simulink model "circuit_Rasp_full_2"  (R2018b)
settings: Solver=VariableStepAuto  StartTime=0.0  StopTime=10.0  RelTol=1e-3
libraries: fl_lib x29, nesl_utility x27, pe_lib x20, elec_lib x6
settings Model: Creator=giovannirenda  LastModifiedBy=giovannirenda
settings DebuggingCC: LibraryContextMissingDiagnostic=none
settings SFSimCC: SimUseLocalCustomCode=off
settings RTWCC: RTWUseLocalCustomCode=off

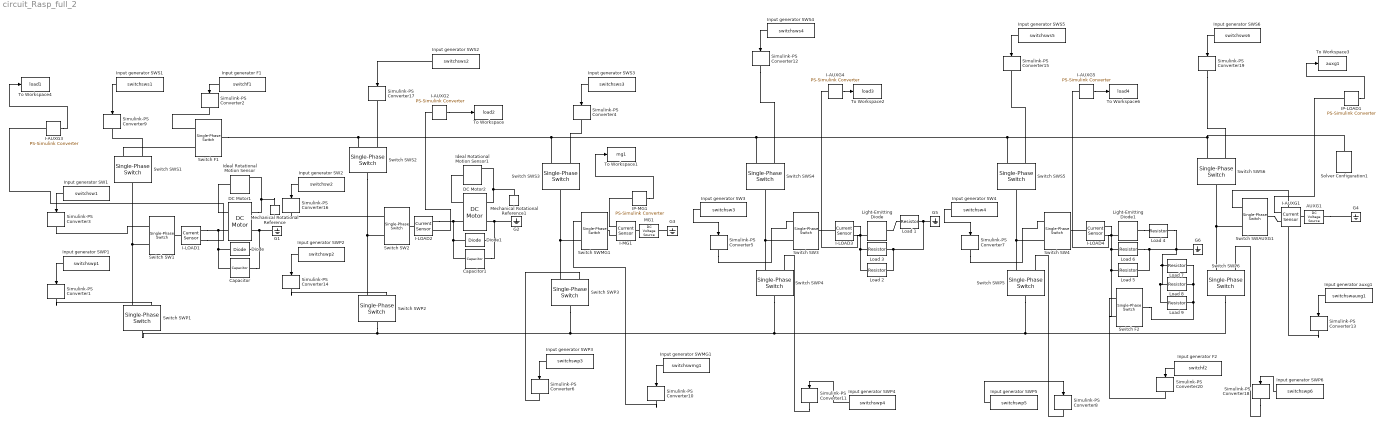
== system circuit_Rasp_full_2 ==
  AUXG1 : fl_lib/Electrical/Electrical Sources/DC Voltage Source  v0=3.3 V
  Capacitor : elec_lib/Passive Devices/Capacitor  enable_table=0  c=10 uF  Cvec=[1e-05, 1e-06] F  Vvec=[0, 10] V  CV_table_symmetry=1  C_tol=5  enable_C_tol=0  tol_distribution=1  nSigma=4  r=1e-6 Ohm  g=0 1/Ohm  enable_operating_limits=0  operating_limit_action=2  max_working_voltage_range=[-25, 25] V  power_rating=1 W  enable_faults=0  fault_action=1  Cscale_faulted=100  R_faulted=1e-3 Ohm  G_faulted=0 1/Ohm  tau_fault=1e-3 s  enable_temporal_fault=0  t_fault=1 s  enable_behavioral_fault=0  max_permissible_voltage_range=[-100, 100] V  t_fail_on_voltage=1 s  i_specify=off  i_priority=None  i=0 A  i_nominal_specify=off  i_nominal_unit=A  i_nominal_value=1  v_specify=off  v_priority=None  v=0 V  v_nominal_specify=off  v_nominal_unit=V  v_nominal_value=1  vc_specify=off  vc_priority=High  vc=0 V  vc_nominal_specify=off  vc_nominal_unit=V  vc_nominal_value=1
  Capacitor1 : elec_lib/Passive Devices/Capacitor  enable_table=0  c=10 uF  Cvec=[1e-05, 1e-06] F  Vvec=[0, 10] V  CV_table_symmetry=1  C_tol=5  enable_C_tol=0  tol_distribution=1  nSigma=4  r=1e-6 Ohm  g=0 1/Ohm  enable_operating_limits=0  operating_limit_action=2  max_working_voltage_range=[-25, 25] V  power_rating=1 W  enable_faults=0  fault_action=1  Cscale_faulted=100  R_faulted=1e-3 Ohm  G_faulted=0 1/Ohm  tau_fault=1e-3 s  enable_temporal_fault=0  t_fault=1 s  enable_behavioral_fault=0  max_permissible_voltage_range=[-100, 100] V  t_fail_on_voltage=1 s  i_specify=off  i_priority=None  i=0 A  i_nominal_specify=off  i_nominal_unit=A  i_nominal_value=1  v_specify=off  v_priority=None  v=0 V  v_nominal_specify=off  v_nominal_unit=V  v_nominal_value=1  vc_specify=off  vc_priority=High  vc=0 V  vc_nominal_specify=off  vc_nominal_unit=V  vc_nominal_value=1
  DC Motor1 : elec_lib/Actuators & Drivers/Rotational Actuators/DC Motor  parameterization=1  Ra=12.7 Ohm  La=12e-6 H  emf_or_torque=1  Kv=0.072e-3 V/rpm  Ki=6.876e-4 N*m/A  T_stall=0.24e-3 N*m  w_max=19100 rpm  w_rated=15000 rpm  P_rated=0.08 W  V_rated=1.5 V  J=0.01 g*cm^2  lam_param=1  lam=0 N*m/(rad/s)  i_noload=0 A  V_i_noload=1.5 V  speed0=0 rpm  alpha=3.93e-3 1/K  Tmeas=25 degC  thermal_mass=100 J/K  initial_temperature=25 degC
  DC Motor2 : elec_lib/Actuators & Drivers/Rotational Actuators/DC Motor  parameterization=1  Ra=12.7 Ohm  La=12e-6 H  emf_or_torque=1  Kv=0.072e-3 V/rpm  Ki=6.876e-4 N*m/A  T_stall=0.24e-3 N*m  w_max=19100 rpm  w_rated=15000 rpm  P_rated=0.08 W  V_rated=1.5 V  J=0.01 g*cm^2  lam_param=1  lam=0 N*m/(rad/s)  i_noload=0 A  V_i_noload=1.5 V  speed0=0 rpm  alpha=3.93e-3 1/K  Tmeas=25 degC  thermal_mass=100 J/K  initial_temperature=25 degC
  Diode : fl_lib/Electrical/Electrical Elements/Diode  Vf=0.6 V  Ron=0.3 Ohm  Goff=1e-8 1/Ohm  i_specify=off  i_priority=None  i=0 A  i_nominal_specify=off  i_nominal_unit=A  i_nominal_value=1  v_specify=off  v_priority=None  v=0 V  v_nominal_specify=off  v_nominal_unit=V  v_nominal_value=1
  Diode1 : fl_lib/Electrical/Electrical Elements/Diode  Vf=0.6 V  Ron=0.3 Ohm  Goff=1e-8 1/Ohm  i_specify=off  i_priority=None  i=0 A  i_nominal_specify=off  i_nominal_unit=A  i_nominal_value=1  v_specify=off  v_priority=None  v=0 V  v_nominal_specify=off  v_nominal_unit=V  v_nominal_value=1
  G{1..6} (6 alike) : fl_lib/Electrical/Electrical Elements/Electrical Reference
  I-AUXG1 : fl_lib/Electrical/Electrical Sensors/Current Sensor
  I-AUXG{2..5} (4 alike) : nesl_utility/PS-Simulink Converter  PhysicalDomain=network_engine_domain  SubClassName=ps_output  LeftPortType=input  RightPortType=output  PseudoPeriodic=off  Frequencies=[]  Unit=A  AffineConversion=off
  I-LOAD{1..4} (4 alike) : fl_lib/Electrical/Electrical Sensors/Current Sensor
  I-MG1 : fl_lib/Electrical/Electrical Sensors/Current Sensor
  IP-LOAD1 : nesl_utility/PS-Simulink Converter  PhysicalDomain=network_engine_domain  SubClassName=ps_output  LeftPortType=input  RightPortType=output  PseudoPeriodic=off  Frequencies=[]  Unit=A  AffineConversion=off
  IP-MG1 : nesl_utility/PS-Simulink Converter  PhysicalDomain=network_engine_domain  SubClassName=ps_output  LeftPortType=input  RightPortType=output  PseudoPeriodic=off  Frequencies=[]  Unit=A  AffineConversion=off
  Ideal Rotational Motion Sensor : fl_lib/Mechanical/Mechanical Sensors/Ideal Rotational Motion Sensor  offset=0 rad
  Ideal Rotational Motion Sensor1 : fl_lib/Mechanical/Mechanical Sensors/Ideal Rotational Motion Sensor  offset=0 rad
  Input generator F1 : FromWorkspace  VariableName=switchf1  SampleTime=1
  Input generator F2 : FromWorkspace  VariableName=switchf2  SampleTime=1
  Input generator SW1 : FromWorkspace  VariableName=switchsw1  SampleTime=1
  Input generator SW2 : FromWorkspace  VariableName=switchsw2  SampleTime=1
  Input generator SW3 : FromWorkspace  VariableName=switchsw3  SampleTime=1
  Input generator SW4 : FromWorkspace  VariableName=switchsw4  SampleTime=1
  Input generator SWMG1 : FromWorkspace  VariableName=switchswmg1  SampleTime=1
  Input generator SWP1 : FromWorkspace  VariableName=switchswp1  SampleTime=1
  Input generator SWP2 : FromWorkspace  VariableName=switchswp2  SampleTime=1
  Input generator SWP3 : FromWorkspace  VariableName=switchswp3  SampleTime=1
  Input generator SWP4 : FromWorkspace  VariableName=switchswp4  SampleTime=1
  Input generator SWP5 : FromWorkspace  VariableName=switchswp5  SampleTime=1
  Input generator SWP6 : FromWorkspace  VariableName=switchswp6  SampleTime=1
  Input generator SWS1 : FromWorkspace  VariableName=switchsws1  SampleTime=1
  Input generator SWS2 : FromWorkspace  VariableName=switchsws2  SampleTime=1
  Input generator SWS3 : FromWorkspace  VariableName=switchsws3  SampleTime=1
  Input generator SWS4 : FromWorkspace  VariableName=switchsws4  SampleTime=1
  Input generator SWS5 : FromWorkspace  VariableName=switchsws5  SampleTime=1
  Input generator SWS6 : FromWorkspace  VariableName=switchsws6  SampleTime=1
  Input generator auxg1 : FromWorkspace  VariableName=switchswauxg1  SampleTime=1
  Light-Emitting Diode : elec_lib/Sensors/Light-Emitting Diode  Gain=0.005 W/A  prmExp=1  I12=[.0017, .003] A  V12=[.9, 1.05] V  IS=5e-5 A  ec=10  RS=0.1 Ohm  Tmeas=25 degC  C_param=1  CJ0=20 pF  VJ=1 V  Mgrad=0.5  Vvec=[.1, 10, 100] V  Cvec=[15, 10, 2] pF  FC=0.5  T_param=1  IS_T2=1.8e-4 A  I1_T2=0.0034 A  V1_T2=1.05 V  Tmeas2=125 degC  EG_param=1  EG=1.11 eV  XTI_param=1  XTI=3  Tdevice=25 degC  i_capacitor_specify=off  i_capacitor_priority=High  i_capacitor=0 A  i_capacitor_nominal_specify=off  i_capacitor_nominal_unit=A  i_capacitor_nominal_value=1  v_capacitor_specify=off  v_capacitor_priority=None  v_capacitor=0 V  v_capacitor_nominal_specify=off  v_capacitor_nominal_unit=V  v_capacitor_nominal_value=1  Rth=[0, 10] K/W  thermal_mass_parameterization=1  thermal_mass=[0, 1] J/K  thermal_time_constant=[0, 10] s  thermal_mass_initial_temperatures=[25, 25] degC
      settings: SourceProductName=Simscape Electronics  SourceProductBaseCode=SN
  Light-Emitting Diode1 : elec_lib/Sensors/Light-Emitting Diode  Gain=0.005 W/A  prmExp=1  I12=[.0017, .003] A  V12=[.9, 1.05] V  IS=5e-5 A  ec=10  RS=0.1 Ohm  Tmeas=25 degC  C_param=1  CJ0=20 pF  VJ=1 V  Mgrad=0.5  Vvec=[.1, 10, 100] V  Cvec=[15, 10, 2] pF  FC=0.5  T_param=1  IS_T2=1.8e-4 A  I1_T2=0.0034 A  V1_T2=1.05 V  Tmeas2=125 degC  EG_param=1  EG=1.11 eV  XTI_param=1  XTI=3  Tdevice=25 degC  i_capacitor_specify=off  i_capacitor_priority=High  i_capacitor=0 A  i_capacitor_nominal_specify=off  i_capacitor_nominal_unit=A  i_capacitor_nominal_value=1  v_capacitor_specify=off  v_capacitor_priority=None  v_capacitor=0 V  v_capacitor_nominal_specify=off  v_capacitor_nominal_unit=V  v_capacitor_nominal_value=1  Rth=[0, 10] K/W  thermal_mass_parameterization=1  thermal_mass=[0, 1] J/K  thermal_time_constant=[0, 10] s  thermal_mass_initial_temperatures=[25, 25] degC
      settings: SourceProductName=Simscape Electronics  SourceProductBaseCode=SN
  Load {1..9} (9 alike) : fl_lib/Electrical/Electrical Elements/Resistor  R=220 Ohm  i_specify=off  i_priority=None  i=0 A  i_nominal_specify=off  i_nominal_unit=A  i_nominal_value=1  v_specify=off  v_priority=None  v=0 V  v_nominal_specify=off  v_nominal_unit=V  v_nominal_value=1
  MG1 : fl_lib/Electrical/Electrical Sources/DC Voltage Source  v0=3.3 V
  Mechanical Rotational Reference : fl_lib/Mechanical/Rotational Elements/Mechanical Rotational Reference
  Mechanical Rotational Reference1 : fl_lib/Mechanical/Rotational Elements/Mechanical Rotational Reference
  Simulink-PS Converter{1..20} (20 alike) : nesl_utility/Simulink-PS Converter  PhysicalDomain=network_engine_domain  SubClassName=ps_input  LeftPortType=input  RightPortType=output  PseudoPeriodic=off  Frequencies=[]  NoiseDistribution=none  NoiseParameters=[]  Unit=1  AffineConversion=off  FilteringAndDerivatives=zero  SimscapeFilterOrder=1  InputFilterTimeConstant=0.001  UdotUserProvided=1
  Solver Configuration1 : nesl_utility/Solver Configuration  PhysicalDomain=network_engine_domain  SubClassName=solver  LeftPortType=input  RightPortType=generic  Tones=[]  Harmonics=[]  SimulateNoise=off  Profile=off  UseLocalSampling=off  EnableSwitchedLinearOptims=on  FrequencyDomain=off  UseCCode=off  RelTol=0.001  AbsTol=1e-06  MinStep=1e-09  ToWorkspace=off  RevertToSquareIcSolve=off  NumHomotopyIterations=100  PhasorMode=off  PhasorModeNumHarmonics=1  DoDC=off  ResidualTolerance=1e-09  UseLocalSolver=off  LocalSolverChoice=NE_BACKWARD_EULER_ADVANCER  LocalSolverSampleTime=0.001  DoFixedCost=off  MaxNonlinIter=3  MaxModeIter=2  LinearAlgebra=Sparse  EquationFormulation=NE_TIME_EF  DelaysMemoryBudget=1024  AutomaticFiltering=on  FilteringTimeConstant=0.001  PartitionStorageMethod=AS_NEEDED  PartitionMemoryBudget=1024
  Switch F1 : pe_lib/Switches & Breakers/Fundamental Components/Single-Phase Switch  R_closed=0.001 Ohm  G_open=1e-6 1/Ohm  threshold=0 V
      settings: SourceProductName=Simscape Electrical  SourceProductBaseCode=PS
  Switch F2 : pe_lib/Switches & Breakers/Fundamental Components/Single-Phase Switch  R_closed=0.001 Ohm  G_open=1e-6 1/Ohm  threshold=0 V
      settings: SourceProductName=Simscape Electrical  SourceProductBaseCode=PS
  Switch SW{1..4} (4 alike) : pe_lib/Switches & Breakers/Fundamental Components/Single-Phase Switch  R_closed=0.001 Ohm  G_open=1e-6 1/Ohm  threshold=0 V
      settings: SourceProductName=Simscape Electrical  SourceProductBaseCode=PS
  Switch SWAUXG1 : pe_lib/Switches & Breakers/Fundamental Components/Single-Phase Switch  R_closed=0.001 Ohm  G_open=1e-6 1/Ohm  threshold=0 V
      settings: SourceProductName=Simscape Electrical  SourceProductBaseCode=PS
  Switch SWMG1 : pe_lib/Switches & Breakers/Fundamental Components/Single-Phase Switch  R_closed=0.001 Ohm  G_open=1e-6 1/Ohm  threshold=0 V
      settings: SourceProductName=Simscape Electrical  SourceProductBaseCode=PS
  Switch SWP{1..6} (6 alike) : pe_lib/Switches & Breakers/Fundamental Components/Single-Phase Switch  R_closed=0.001 Ohm  G_open=1e-6 1/Ohm  threshold=0 V
      settings: SourceProductName=Simscape Electrical  SourceProductBaseCode=PS
  Switch SWS{1..6} (6 alike) : pe_lib/Switches & Breakers/Fundamental Components/Single-Phase Switch  R_closed=0.001 Ohm  G_open=1e-6 1/Ohm  threshold=0 V
      settings: SourceProductName=Simscape Electrical  SourceProductBaseCode=PS
  To Workspace : ToWorkspace  VariableName=load2  SampleTime=1
      settings: Save2DSignal=2-D array (concatenate along first dimension)
  To Workspace1 : ToWorkspace  VariableName=mg1  SampleTime=1
      settings: Save2DSignal=2-D array (concatenate along first dimension)
  To Workspace2 : ToWorkspace  VariableName=load3  SampleTime=1
      settings: Save2DSignal=2-D array (concatenate along first dimension)
  To Workspace3 : ToWorkspace  VariableName=auxg1  SampleTime=1
      settings: Save2DSignal=2-D array (concatenate along first dimension)
  To Workspace4 : ToWorkspace  VariableName=load1  SampleTime=1
      settings: Save2DSignal=2-D array (concatenate along first dimension)
  To Workspace6 : ToWorkspace  VariableName=load4  SampleTime=1
  wires:
  Input generator SWS1/1 -> Simulink-PS Converter9/1
  Input generator SWP1/1 -> Simulink-PS Converter1/1
  Input generator F1/1 -> Simulink-PS Converter2/1
  Input generator SW1/1 -> Simulink-PS Converter3/1
  Input generator SWS3/1 -> Simulink-PS Converter4/1
  Input generator SWP3/1 -> Simulink-PS Converter6/1
  Input generator SWMG1/1 -> Simulink-PS Converter10/1
  I-AUXG3/1 -> To Workspace4/1
  IP-MG1/1 -> To Workspace1/1
  IP-LOAD1/1 -> To Workspace3/1
  Input generator auxg1/1 -> Simulink-PS Converter13/1
  Input generator SWP2/1 -> Simulink-PS Converter14/1
  Input generator SW2/1 -> Simulink-PS Converter16/1
  Input generator SWS2/1 -> Simulink-PS Converter17/1
  I-AUXG2/1 -> To Workspace/1
  I-AUXG4/1 -> To Workspace2/1
  Input generator SWS4/1 -> Simulink-PS Converter12/1
  Input generator SWP4/1 -> Simulink-PS Converter11/1
  Input generator SW3/1 -> Simulink-PS Converter5/1
  Input generator SW4/1 -> Simulink-PS Converter7/1
  Input generator SWP5/1 -> Simulink-PS Converter8/1
  Input generator SWS5/1 -> Simulink-PS Converter15/1
  I-AUXG5/1 -> To Workspace6/1
  Input generator SWP6/1 -> Simulink-PS Converter18/1
  Input generator SWS6/1 -> Simulink-PS Converter19/1
  Input generator F2/1 -> Simulink-PS Converter20/1
  connections:
  Switch SW1/LConn2 -- Switch SWP1/LConn2 -- Switch SWS1/RConn1
  Capacitor/RConn1 -- Diode/LConn1 -- G1/LConn1 -- DC Motor1/RConn1
  G3/LConn1 -- MG1/RConn1
  Switch SWS6/LConn2 -- Solver Configuration1/RConn1 -- Switch SWS4/LConn2 -- Switch SWS3/LConn2 -- Switch SWS2/LConn2 -- Switch F1/RConn1 -- Switch SWS5/LConn2
  Switch SWP1/RConn1 -- Switch SWP2/RConn1 -- Switch SWP6/RConn1 -- Switch SWP5/RConn1 -- Switch SWP4/RConn1 -- Switch SWP3/RConn1
  Switch SWS1/LConn2 -- Switch F1/LConn2
  Switch SWS1/LConn1 -- Simulink-PS Converter9/RConn1
  Simulink-PS Converter1/RConn1 -- Switch SWP1/LConn1
  Simulink-PS Converter2/RConn1 -- Switch F1/LConn1
  Simulink-PS Converter3/RConn1 -- Switch SW1/LConn1
  Switch SWS3/LConn1 -- Simulink-PS Converter4/RConn1
  Simulink-PS Converter6/RConn1 -- Switch SWP3/LConn1
  Simulink-PS Converter10/RConn1 -- Switch SWMG1/LConn1
  I-LOAD1/RConn1 -- I-AUXG3/LConn1
  I-MG1/RConn2 -- Switch SWMG1/RConn1
  I-MG1/LConn1 -- MG1/LConn1
  I-LOAD1/LConn1 -- Switch SW1/RConn1
  IP-MG1/LConn1 -- I-MG1/RConn1
  I-AUXG1/LConn1 -- AUXG1/LConn1
  AUXG1/RConn1 -- G4/LConn1
  Switch SWAUXG1/RConn1 -- I-AUXG1/RConn2
  IP-LOAD1/LConn1 -- I-AUXG1/RConn1
  Simulink-PS Converter13/RConn1 -- Switch SWAUXG1/LConn1
  Diode/RConn1 -- Capacitor/LConn1 -- I-LOAD1/RConn2 -- DC Motor1/LConn1
  Switch SWS2/RConn1 -- Switch SW2/LConn2 -- Switch SWP2/LConn2
  Capacitor1/RConn1 -- Diode1/LConn1 -- G2/LConn1 -- DC Motor2/RConn1
  DC Motor2/LConn1 -- I-LOAD2/RConn2 -- Diode1/RConn1 -- Capacitor1/LConn1
  Switch SW2/LConn1 -- Simulink-PS Converter16/RConn1
  Switch SWS2/LConn1 -- Simulink-PS Converter17/RConn1
  I-LOAD2/LConn1 -- Switch SW2/RConn1
  I-AUXG2/LConn1 -- I-LOAD2/RConn1
  Simulink-PS Converter14/RConn1 -- Switch SWP2/LConn1
  Switch SWMG1/LConn2 -- Switch SWS3/RConn1 -- Switch SWP3/LConn2
  Switch SWP4/LConn2 -- Switch SWS4/RConn1 -- Switch SW3/LConn2
  G5/LConn1 -- Load 2/RConn1 -- Load 3/RConn1 -- Load 1/RConn1
  I-LOAD3/LConn1 -- Switch SW3/RConn1
  Load 2/LConn1 -- Load 3/LConn1 -- I-LOAD3/RConn2 -- Light-Emitting Diode/LConn2
  I-LOAD3/RConn1 -- I-AUXG4/LConn1
  Simulink-PS Converter12/RConn1 -- Switch SWS4/LConn1
  Simulink-PS Converter11/RConn1 -- Switch SWP4/LConn1
  Simulink-PS Converter5/RConn1 -- Switch SW3/LConn1
  Switch SWP5/LConn2 -- Switch SWS5/RConn1 -- Switch SW4/LConn2
  Load 9/LConn1 -- Load 4/RConn1 -- G6/LConn1 -- Load 6/RConn1 -- Load 5/RConn1 -- Load 7/LConn1 -- Load 8/LConn1
  Light-Emitting Diode1/LConn2 -- I-LOAD4/RConn2 -- Switch F2/LConn2 -- Load 5/LConn1 -- Load 6/LConn1
  Simulink-PS Converter7/RConn1 -- Switch SW4/LConn1
  I-LOAD4/LConn1 -- Switch SW4/RConn1
  Simulink-PS Converter8/RConn1 -- Switch SWP5/LConn1
  Switch SWS5/LConn1 -- Simulink-PS Converter15/RConn1
  I-LOAD4/RConn1 -- I-AUXG5/LConn1
  Switch SWAUXG1/LConn2 -- Switch SWS6/RConn1 -- Switch SWP6/LConn2
  Light-Emitting Diode/RConn1 -- Load 1/LConn1
  Light-Emitting Diode1/RConn1 -- Load 4/LConn1
  Simulink-PS Converter18/RConn1 -- Switch SWP6/LConn1
  Simulink-PS Converter19/RConn1 -- Switch SWS6/LConn1
  Load 7/RConn1 -- Switch F2/RConn1 -- Load 9/RConn1 -- Load 8/RConn1
  Simulink-PS Converter20/RConn1 -- Switch F2/LConn1
  Ideal Rotational Motion Sensor/LConn1 -- DC Motor1/LConn2
  DC Motor2/LConn2 -- Ideal Rotational Motion Sensor1/LConn1
  DC Motor2/RConn2 -- Mechanical Rotational Reference1/LConn1 -- Ideal Rotational Motion Sensor1/RConn1
  DC Motor1/RConn2 -- Mechanical Rotational Reference/LConn1 -- Ideal Rotational Motion Sensor/RConn1
